simulink model "plant_model"  (R2021a)
settings: Solver=VariableStepAuto  StartTime=0.0  StopTime=10.0  RelTol=1e-3
settings Model: Creator=furkan  LastModifiedBy=furkan

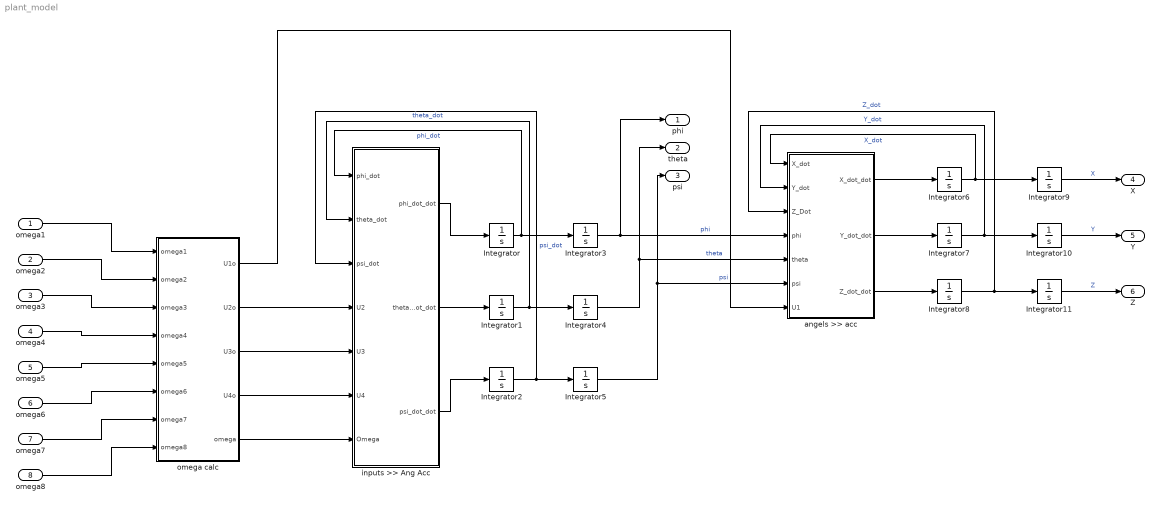
== system plant_model ==
  omega1 : Inport
  omega2 : Inport  Port=2
  omega3 : Inport  Port=3
  omega4 : Inport  Port=4
  omega5 : Inport  Port=5
  omega6 : Inport  Port=6
  omega7 : Inport  Port=7
  omega8 : Inport  Port=8
  Integrator{,1..11} (12 alike) : Integrator
  angels >> acc : Subsystem
  inputs >> Ang Acc : Subsystem
  omega calc : Subsystem
  phi : Outport
  theta : Outport  Port=2
  psi : Outport  Port=3
  X : Outport  Port=4
  Y : Outport  Port=5
  Z : Outport  Port=6
  wires:
  omega1/1 -> omega calc/1(omega1)
  omega2/1 -> omega calc/2(omega2)
  omega3/1 -> omega calc/3(omega3)
  omega4/1 -> omega calc/4(omega4)
  omega5/1 -> omega calc/5(omega5)
  omega6/1 -> omega calc/6(omega6)
  omega7/1 -> omega calc/7(omega7)
  omega8/1 -> omega calc/8(omega8)
  omega calc/2(U2o) -> inputs >> Ang Acc/4(U2)
  omega calc/3(U3o) -> inputs >> Ang Acc/5(U3)
  omega calc/4(U4o) -> inputs >> Ang Acc/6(U4)
  omega calc/5(omega) -> inputs >> Ang Acc/7(Omega)
  inputs >> Ang Acc/1(phi_dot_dot) -> Integrator/1
  inputs >> Ang Acc/2(theta_dot_dot) -> Integrator1/1
  inputs >> Ang Acc/3(psi_dot_dot) -> Integrator2/1
  Integrator/1 -> Integrator3/1, inputs >> Ang Acc/1(phi_dot)  "phi_dot"
  Integrator1/1 -> Integrator4/1, inputs >> Ang Acc/2(theta_dot)  "theta_dot"
  Integrator2/1 -> Integrator5/1, inputs >> Ang Acc/3(psi_dot)  "psi_dot"
  Integrator3/1 -> angels >> acc/4(phi), phi/1  "phi"
  Integrator4/1 -> angels >> acc/5(theta), theta/1  "theta"
  Integrator5/1 -> angels >> acc/6(psi), psi/1  "psi"
  omega calc/1(U1o) -> angels >> acc/7(U1)
  angels >> acc/1(X_dot_dot) -> Integrator6/1
  angels >> acc/2(Y_dot_dot) -> Integrator7/1
  angels >> acc/3(Z_dot_dot) -> Integrator8/1
  Integrator6/1 -> angels >> acc/1(X_dot), Integrator9/1  "X_dot"
  Integrator7/1 -> Integrator10/1, angels >> acc/2(Y_dot)  "Y_dot"
  Integrator8/1 -> angels >> acc/3(Z_Dot), Integrator11/1  "Z_dot"
  Integrator9/1 -> X/1  "X"
  Integrator10/1 -> Y/1  "Y"
  Integrator11/1 -> Z/1  "Z"

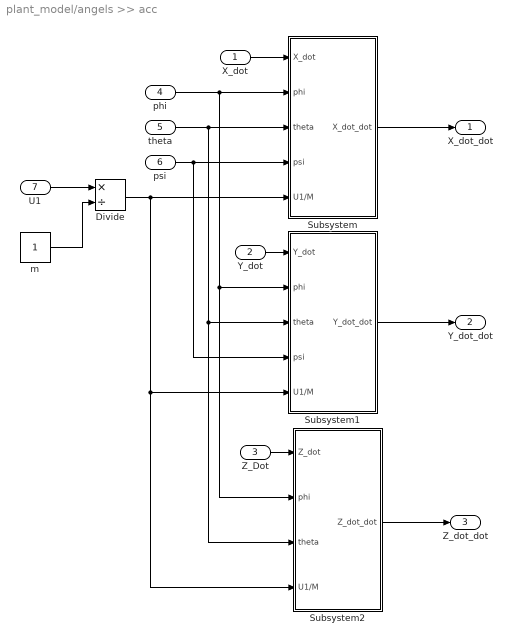
== system plant_model/angels >> acc ==
  X_dot : Inport
  Y_dot : Inport  Port=2
  Z_Dot : Inport  Port=3
  phi : Inport  Port=4
  theta : Inport  Port=5
  psi : Inport  Port=6
  U1 : Inport  Port=7
  Divide : Product  Inputs=*/
  Subsystem : Subsystem
  Subsystem1 : Subsystem
  Subsystem2 : Subsystem
  m : Constant
  X_dot_dot : Outport
  Y_dot_dot : Outport  Port=2
  Z_dot_dot : Outport  Port=3
  wires:
  U1/1 -> Divide/1
  m/1 -> Divide/2
  X_dot/1 -> Subsystem/1(X_dot)
  phi/1 -> Subsystem2/2(phi), Subsystem1/2(phi), Subsystem/2(phi)
  theta/1 -> Subsystem2/3(theta), Subsystem1/3(theta), Subsystem/3(theta)
  psi/1 -> Subsystem1/4(psi), Subsystem/4(psi)
  Divide/1 -> Subsystem2/4(U1/M), Subsystem1/5(U1/M), Subsystem/5(U1/M)
  Subsystem/1(X_dot_dot) -> X_dot_dot/1
  Y_dot/1 -> Subsystem1/1(Y_dot)
  Z_Dot/1 -> Subsystem2/1(Z_dot)
  Subsystem1/1(Y_dot_dot) -> Y_dot_dot/1
  Subsystem2/1(Z_dot_dot) -> Z_dot_dot/1

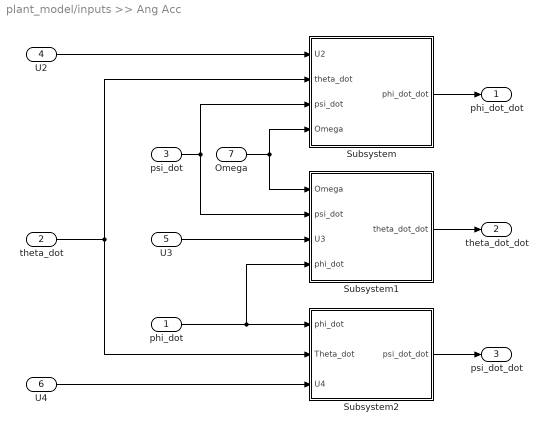
== system plant_model/inputs >> Ang Acc ==
  phi_dot : Inport
  theta_dot : Inport  Port=2
  psi_dot : Inport  Port=3
  U2 : Inport  Port=4
  U3 : Inport  Port=5
  U4 : Inport  Port=6
  Omega : Inport  Port=7
  Subsystem : Subsystem
  Subsystem1 : Subsystem
  Subsystem2 : Subsystem
  phi_dot_dot : Outport
  theta_dot_dot : Outport  Port=2
  psi_dot_dot : Outport  Port=3
  wires:
  Subsystem/1(phi_dot_dot) -> phi_dot_dot/1
  Subsystem2/1(psi_dot_dot) -> psi_dot_dot/1
  Subsystem1/1(theta_dot_dot) -> theta_dot_dot/1
  Omega/1 -> Subsystem1/1(Omega), Subsystem/4(Omega)
  psi_dot/1 -> Subsystem/3(psi_dot), Subsystem1/2(psi_dot)
  U3/1 -> Subsystem1/3(U3)
  phi_dot/1 -> Subsystem1/4(phi_dot), Subsystem2/1(phi_dot)
  theta_dot/1 -> Subsystem2/2(Theta_dot), Subsystem/2(theta_dot)
  U2/1 -> Subsystem/1(U2)
  U4/1 -> Subsystem2/3(U4)

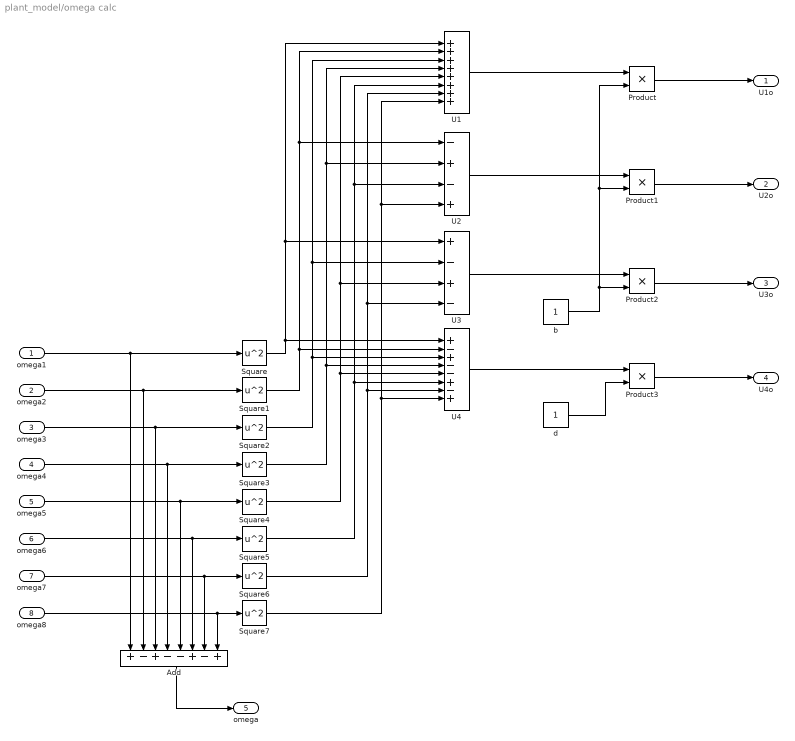
== system plant_model/omega calc ==
  omega1 : Inport
  omega2 : Inport  Port=2
  omega3 : Inport  Port=3
  omega4 : Inport  Port=4
  omega5 : Inport  Port=5
  omega6 : Inport  Port=6
  omega7 : Inport  Port=7
  omega8 : Inport  Port=8
  Add : Sum  Inputs=+-+--+-+
  Product{,1..3} (4 alike) : Product
  Square{,1..7} (8 alike) : Math  Operator=square  SaturateOnIntegerOverflow=on
  U1 : Sum  Inputs=++++++++
  U2 : Sum  Inputs=-+-+
  U3 : Sum  Inputs=+-+-
  U4 : Sum  Inputs=+-+--+-+
  b : Constant
  d : Constant
  U1o : Outport
  U2o : Outport  Port=2
  U3o : Outport  Port=3
  U4o : Outport  Port=4
  omega : Outport  Port=5
  wires:
  Square6/1 -> U1/7, U3/4, U4/7
  U3/1 -> Product2/1
  omega6/1 -> Square5/1, Add/6
  Square5/1 -> U4/6, U1/6, U2/3
  omega7/1 -> Square6/1, Add/7
  Product2/1 -> U3o/1
  Product1/1 -> U2o/1
  Square4/1 -> U4/5, U1/5, U3/3
  Square3/1 -> U4/4, U1/4, U2/2
  Square/1 -> U4/1, U3/1, U1/1
  b/1 -> Product/2, Product1/2, Product2/2
  omega1/1 -> Square/1, Add/1
  U1/1 -> Product/1
  omega8/1 -> Add/8, Square7/1
  Add/1 -> omega/1
  Square7/1 -> U1/8, U2/4, U4/8
  d/1 -> Product3/2
  omega2/1 -> Add/2, Square1/1
  Square2/1 -> U4/3, U3/2, U1/3
  Product/1 -> U1o/1
  U4/1 -> Product3/1
  Square1/1 -> U4/2, U1/2, U2/1
  omega3/1 -> Square2/1, Add/3
  omega5/1 -> Add/5, Square4/1
  U2/1 -> Product1/1
  omega4/1 -> Square3/1, Add/4
  Product3/1 -> U4o/1

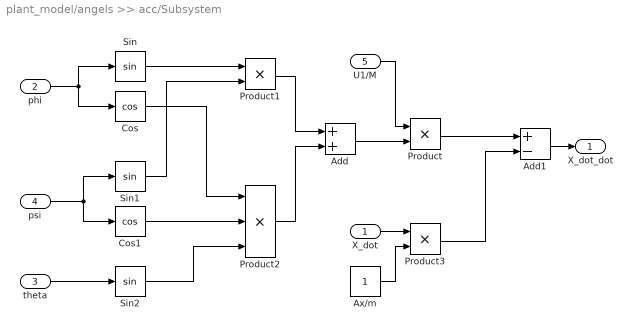
== system plant_model/angels >> acc/Subsystem ==
  X_dot : Inport
  phi : Inport  Port=2
  theta : Inport  Port=3
  psi : Inport  Port=4
  U1/M : Inport  Port=5
  Add : Sum
  Add1 : Sum  Inputs=+-
  Ax/m : Constant
  Cos : Trigonometry  Operator=cos
  Cos1 : Trigonometry  Operator=cos
  Product : Product
  Product1 : Product
  Product2 : Product  Inputs=3
  Product3 : Product
  Sin : Trigonometry
  Sin1 : Trigonometry
  Sin2 : Trigonometry
  X_dot_dot : Outport
  wires:
  U1/M/1 -> Product/1
  phi/1 -> Cos/1, Sin/1
  psi/1 -> Sin1/1, Cos1/1
  theta/1 -> Sin2/1
  Sin/1 -> Product1/1
  Sin1/1 -> Product1/2
  Cos/1 -> Product2/1
  Cos1/1 -> Product2/2
  Sin2/1 -> Product2/3
  Product1/1 -> Add/1
  Product2/1 -> Add/2
  Add/1 -> Product/2
  X_dot/1 -> Product3/1
  Ax/m/1 -> Product3/2
  Product/1 -> Add1/1
  Product3/1 -> Add1/2
  Add1/1 -> X_dot_dot/1

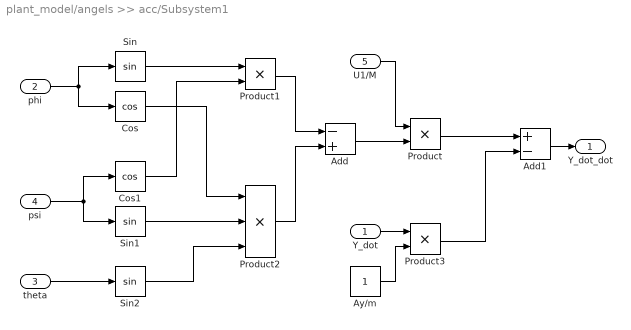
== system plant_model/angels >> acc/Subsystem1 ==
  Y_dot : Inport
  phi : Inport  Port=2
  theta : Inport  Port=3
  psi : Inport  Port=4
  U1/M : Inport  Port=5
  Add : Sum  Inputs=-+
  Add1 : Sum  Inputs=+-
  Ay/m : Constant
  Cos : Trigonometry  Operator=cos
  Cos1 : Trigonometry  Operator=cos
  Product : Product
  Product1 : Product
  Product2 : Product  Inputs=3
  Product3 : Product
  Sin : Trigonometry
  Sin1 : Trigonometry
  Sin2 : Trigonometry
  Y_dot_dot : Outport
  wires:
  U1/M/1 -> Product/1
  phi/1 -> Cos/1, Sin/1
  psi/1 -> Sin1/1, Cos1/1
  theta/1 -> Sin2/1
  Sin/1 -> Product1/1
  Cos/1 -> Product2/1
  Sin2/1 -> Product2/3
  Product1/1 -> Add/1
  Product2/1 -> Add/2
  Add/1 -> Product/2
  Y_dot/1 -> Product3/1
  Ay/m/1 -> Product3/2
  Product/1 -> Add1/1
  Product3/1 -> Add1/2
  Add1/1 -> Y_dot_dot/1
  Cos1/1 -> Product1/2
  Sin1/1 -> Product2/2

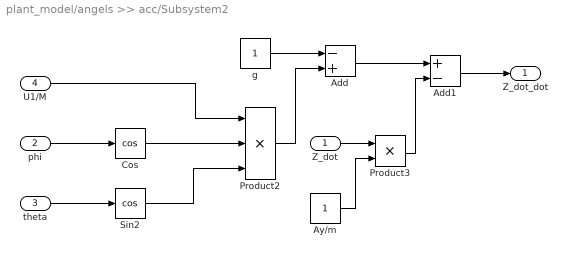
== system plant_model/angels >> acc/Subsystem2 ==
  Z_dot : Inport
  phi : Inport  Port=2
  theta : Inport  Port=3
  U1/M : Inport  Port=4
  Add : Sum  Inputs=-+
  Add1 : Sum  Inputs=+-
  Ay/m : Constant
  Cos : Trigonometry  Operator=cos
  Product2 : Product  Inputs=3
  Product3 : Product
  Sin2 : Trigonometry  Operator=cos
  g : Constant
  Z_dot_dot : Outport
  wires:
  phi/1 -> Cos/1
  theta/1 -> Sin2/1
  Sin2/1 -> Product2/3
  g/1 -> Add/1
  Product2/1 -> Add/2
  Z_dot/1 -> Product3/1
  Ay/m/1 -> Product3/2
  Add/1 -> Add1/1
  Product3/1 -> Add1/2
  Add1/1 -> Z_dot_dot/1
  Cos/1 -> Product2/2
  U1/M/1 -> Product2/1

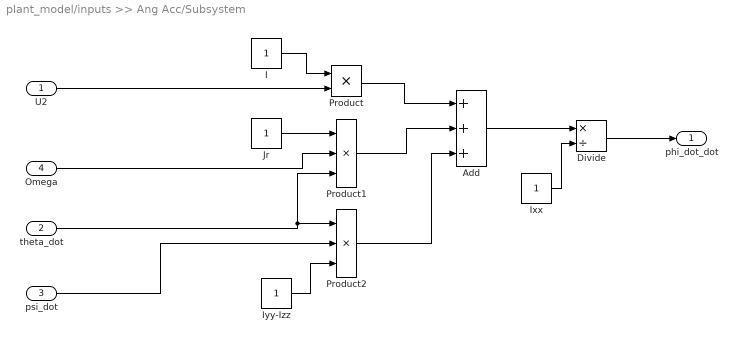
== system plant_model/inputs >> Ang Acc/Subsystem ==
  U2 : Inport
  theta_dot : Inport  Port=2
  psi_dot : Inport  Port=3
  Omega : Inport  Port=4
  Add : Sum  Inputs=+++
  Divide : Product  Inputs=*/
  I : Constant
  Ixx : Constant
  Iyy-Izz : Constant
  Jr : Constant
  Product : Product
  Product1 : Product  Inputs=3
  Product2 : Product  Inputs=3
  phi_dot_dot : Outport
  wires:
  Iyy-Izz/1 -> Product2/3
  Add/1 -> Divide/1
  I/1 -> Product/1
  theta_dot/1 -> Product1/3, Product2/1
  Product2/1 -> Add/3
  Product1/1 -> Add/2
  Ixx/1 -> Divide/2
  U2/1 -> Product/2
  Jr/1 -> Product1/1
  Product/1 -> Add/1
  Divide/1 -> phi_dot_dot/1
  Omega/1 -> Product1/2
  psi_dot/1 -> Product2/2

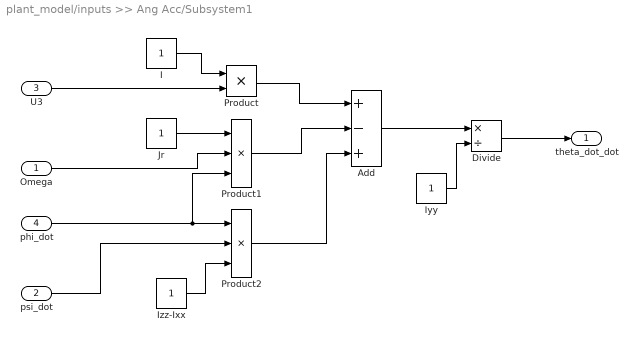
== system plant_model/inputs >> Ang Acc/Subsystem1 ==
  Omega : Inport
  psi_dot : Inport  Port=2
  U3 : Inport  Port=3
  phi_dot : Inport  Port=4
  Add : Sum  Inputs=+-+
  Divide : Product  Inputs=*/
  I : Constant
  Iyy : Constant
  Izz-Ixx : Constant
  Jr : Constant
  Product : Product
  Product1 : Product  Inputs=3
  Product2 : Product  Inputs=3
  theta_dot_dot : Outport
  wires:
  Izz-Ixx/1 -> Product2/3
  Add/1 -> Divide/1
  I/1 -> Product/1
  phi_dot/1 -> Product1/3, Product2/1
  Product2/1 -> Add/3
  Product1/1 -> Add/2
  Iyy/1 -> Divide/2
  U3/1 -> Product/2
  Jr/1 -> Product1/1
  Product/1 -> Add/1
  Divide/1 -> theta_dot_dot/1
  Omega/1 -> Product1/2
  psi_dot/1 -> Product2/2

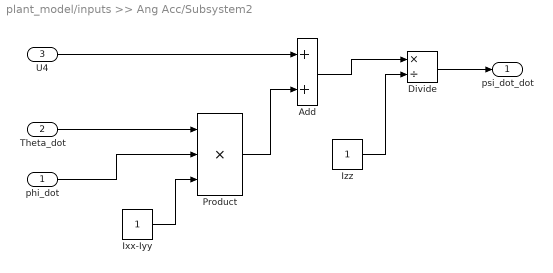
== system plant_model/inputs >> Ang Acc/Subsystem2 ==
  phi_dot : Inport
  Theta_dot : Inport  Port=2
  U4 : Inport  Port=3
  Add : Sum
  Divide : Product  Inputs=*/
  Ixx-Iyy : Constant
  Izz : Constant
  Product : Product  Inputs=3
  psi_dot_dot : Outport
  wires:
  Product/1 -> Add/2
  Divide/1 -> psi_dot_dot/1
  Add/1 -> Divide/1
  Izz/1 -> Divide/2
  U4/1 -> Add/1
  Ixx-Iyy/1 -> Product/3
  phi_dot/1 -> Product/2
  Theta_dot/1 -> Product/1
